simulink library "ammclib_bam_S32K3xx"  (R2016a)
settings: Solver=VariableStepAuto  SolverMode=SingleTasking  StartTime=0.0  StopTime=10.0  RelTol=1e-3
undefined symbols (not defined in the file or in its folder): a1, a2, ADCMaxError, autoCalcEn, b0, b1, b2, cfg, dgain, escale, f16A1, f16A2, f16ADCMaxError, f16B0, f16B1, f16B2, f16C1, f16CC1sc, f16CC1sc_D, f16CC1sc_Q, f16CC2sc, f16CC2sc_D, f16CC2sc_Q, f16DerivGain, f16EGain, f16FiltCoef, f16HystOff, f16HystOn, f16IGain, f16IntegGain, f16IntegGain_D, f16IntegGain_Q, f16IntegGainQ, f16Kd, f16KLs, f16Kq, f16KRs, f16Limit, f16LowerLimit, f16LowerLimit_D, f16LowerLimit_Q, f16LowerLimitQ, f16ModIndex, f16OutValOff, f16OutValOn, f16PropGain, f16PropGain_D, f16PropGain_Q, f16PropGainQ, f16RampDown, f16RampUp, f16UGain, f16UpperLimit, f16UpperLimit_D, f16UpperLimit_Q, f16UpperLimitQ, f16WIGain, f32A1, f32A2, f32ADCMaxError ... (+180)
(part 47 of 50)

== system ammclib_bam_S32K3xx/GFLIB/FLT/GFLIB_ControllerPIpAW_FLT ==
  fltInErr : Inport  OutDataTypeStr=single  SampleTime=SampleTime
  fltControllerPIpAWOut_preset : Inport  Port=2  OutDataTypeStr=single  SampleTime=SampleTime
  Reset : ResetPort  DisableCoverage=on
  GFLIB_ControllerPIpAW_SF : S-Function  FunctionName=GFLIB_ControllerPIpAW_SF_FLT  Parameters=showStates,resetStatesEnable,fltPropGain,fltIntegGain,fltLowerLimit,fltUpperLimit,pgain,igain,lowerLimit,upperLimit,autoCalcEn  SFunctionDeploymentMode=off  EnableBusSupport=off
  copyright : Subsystem
      mask Display: text(10,90,'FILE:');text(10,75,'DESRIPTION:');text(10,60,'COPYRIGHT:');text(10,45,'VERSION:');text(10,30,'DATE:')
  copyright2 : Subsystem
      mask Display: text(10,90,'GFLIB_ControllerPIpAW_BAM_FLT.slx');text(10,75,'Parallel form of a standard PI controller with anti-windup.');text(10,60,'NXP 2022');text(10,45,'1.0');text(10,30,'20-Apr-2022');
  fltInK_1 : Ground
  fltInK_1_Out : Terminator
  fltIntegGain : Ground
  fltIntegPartK_1 : Ground
  fltIntegPartK_1_Out : Terminator
  fltLowerLimit : Ground
  fltPropGain : Ground
  fltUpperLimit : Ground
  fltOut : Outport
  u16LimitFlag : Outport  Port=2
  wires:
  GFLIB_ControllerPIpAW_SF/4 -> fltInK_1_Out/1
  GFLIB_ControllerPIpAW_SF/3 -> fltIntegPartK_1_Out/1
  GFLIB_ControllerPIpAW_SF/2 -> u16LimitFlag/1
  GFLIB_ControllerPIpAW_SF/1 -> fltOut/1
  fltInK_1/1 -> GFLIB_ControllerPIpAW_SF/8
  fltIntegPartK_1/1 -> GFLIB_ControllerPIpAW_SF/7
  fltUpperLimit/1 -> GFLIB_ControllerPIpAW_SF/6
  fltLowerLimit/1 -> GFLIB_ControllerPIpAW_SF/5
  fltIntegGain/1 -> GFLIB_ControllerPIpAW_SF/4
  fltPropGain/1 -> GFLIB_ControllerPIpAW_SF/3
  fltControllerPIpAWOut_preset/1 -> GFLIB_ControllerPIpAW_SF/2
  fltInErr/1 -> GFLIB_ControllerPIpAW_SF/1

== system ammclib_bam_S32K3xx/GFLIB/FLT/GFLIB_ControllerPIp_FLT ==
  fltInErr : Inport  OutDataTypeStr=single  SampleTime=SampleTime
  fltControllerPIpOut_preset : Inport  Port=2  OutDataTypeStr=single  SampleTime=SampleTime
  Reset : ResetPort  DisableCoverage=on
  GFLIB_ControllerPIp_SF : S-Function  FunctionName=GFLIB_ControllerPIp_SF_FLT  Parameters=showStates,resetStatesEnable,fltPropGain,fltIntegGain,pgain,igain,autoCalcEn  SFunctionDeploymentMode=off  EnableBusSupport=off
  copyright : Subsystem
      mask Display: text(10,90,'FILE:');text(10,75,'DESRIPTION:');text(10,60,'COPYRIGHT:');text(10,45,'VERSION:');text(10,30,'DATE:')
  copyright2 : Subsystem
      mask Display: text(10,90,'GFLIB_ControllerPIp_BAM_FLT.slx');text(10,75,'Parallel form of a standard PI controller without anti-windup.');text(10,60,'NXP 2022');text(10,45,'1.0');text(10,30,'20-Apr-2022');
  fltInK_1 : Ground
  fltInK_1_Out : Terminator
  fltIntegGain : Ground
  fltIntegPartK_1 : Ground
  fltIntegPartK_1_Out : Terminator
  fltPropGain : Ground
  fltOut : Outport
  wires:
  GFLIB_ControllerPIp_SF/3 -> fltInK_1_Out/1
  GFLIB_ControllerPIp_SF/2 -> fltIntegPartK_1_Out/1
  GFLIB_ControllerPIp_SF/1 -> fltOut/1
  fltInK_1/1 -> GFLIB_ControllerPIp_SF/6
  fltIntegPartK_1/1 -> GFLIB_ControllerPIp_SF/5
  fltIntegGain/1 -> GFLIB_ControllerPIp_SF/4
  fltPropGain/1 -> GFLIB_ControllerPIp_SF/3
  fltControllerPIpOut_preset/1 -> GFLIB_ControllerPIp_SF/2
  fltInErr/1 -> GFLIB_ControllerPIp_SF/1

== system ammclib_bam_S32K3xx/GFLIB/FLT/GFLIB_ControllerPIrAW_FLT ==
  fltInErr : Inport  OutDataTypeStr=single  SampleTime=SampleTime
  fltControllerPIrAWOut_preset : Inport  Port=2  OutDataTypeStr=single  SampleTime=SampleTime
  Reset : ResetPort  DisableCoverage=on
  GFLIB_ControllerPIrAW_SF : S-Function  FunctionName=GFLIB_ControllerPIrAW_SF_FLT  Parameters=showStates,resetStatesEnable,fltUpperLimit,fltLowerLimit,fltCC1sc,fltCC2sc,intmethod,pgain,igain,upperLimit,lowerLimit,autoCalcEn  SFunctionDeploymentMode=off  EnableBusSupport=off
  copyright : Subsystem
      mask Display: text(10,90,'FILE:');text(10,75,'DESRIPTION:');text(10,60,'COPYRIGHT:');text(10,45,'VERSION:');text(10,30,'DATE:')
  copyright2 : Subsystem
      mask Display: text(10,90,'GFLIB_ControllerPIrAW_BAM_FLT.slx');text(10,75,'Recurrent form PI controller with anti-windup.');text(10,60,'NXP 2022');text(10,45,'1.0');text(10,30,'20-Apr-2022');
  fltAcc : Ground
  fltAcc_Out : Terminator
  fltCC1sc : Ground
  fltCC2sc : Ground
  fltInErrK1 : Ground
  fltInErrK1_Out : Terminator
  fltLowerLimit : Ground
  fltUpperLimit : Ground
  fltOut : Outport
  wires:
  GFLIB_ControllerPIrAW_SF/3 -> fltInErrK1_Out/1
  GFLIB_ControllerPIrAW_SF/2 -> fltAcc_Out/1
  GFLIB_ControllerPIrAW_SF/1 -> fltOut/1
  fltCC2sc/1 -> GFLIB_ControllerPIrAW_SF/8
  fltCC1sc/1 -> GFLIB_ControllerPIrAW_SF/7
  fltInErrK1/1 -> GFLIB_ControllerPIrAW_SF/6
  fltAcc/1 -> GFLIB_ControllerPIrAW_SF/5
  fltLowerLimit/1 -> GFLIB_ControllerPIrAW_SF/4
  fltUpperLimit/1 -> GFLIB_ControllerPIrAW_SF/3
  fltControllerPIrAWOut_preset/1 -> GFLIB_ControllerPIrAW_SF/2
  fltInErr/1 -> GFLIB_ControllerPIrAW_SF/1

== system ammclib_bam_S32K3xx/GFLIB/FLT/GFLIB_ControllerPIr_FLT ==
  fltInErr : Inport  OutDataTypeStr=single  SampleTime=SampleTime
  fltControllerPIrOut_preset : Inport  Port=2  OutDataTypeStr=single  SampleTime=SampleTime
  Reset : ResetPort  DisableCoverage=on
  GFLIB_ControllerPIr_SF : S-Function  FunctionName=GFLIB_ControllerPIr_SF_FLT  Parameters=showStates,resetStatesEnable,fltCC1sc,fltCC2sc,intmethod,pgain,igain,autoCalcEn  SFunctionDeploymentMode=off  EnableBusSupport=off
  copyright : Subsystem
      mask Display: text(10,90,'FILE:');text(10,75,'DESRIPTION:');text(10,60,'COPYRIGHT:');text(10,45,'VERSION:');text(10,30,'DATE:')
  copyright2 : Subsystem
      mask Display: text(10,90,'GFLIB_ControllerPIr_BAM_FLT.slx');text(10,75,'Recurrent form PI controller without anti-windup.');text(10,60,'NXP 2022');text(10,45,'1.0');text(10,30,'20-Apr-2022');
  fltAcc : Ground
  fltAcc_Out : Terminator
  fltCC1sc : Ground
  fltCC2sc : Ground
  fltInErrK1 : Ground
  fltInErrK1_Out : Terminator
  fltOut : Outport
  wires:
  GFLIB_ControllerPIr_SF/3 -> fltInErrK1_Out/1
  GFLIB_ControllerPIr_SF/2 -> fltAcc_Out/1
  GFLIB_ControllerPIr_SF/1 -> fltOut/1
  fltInErrK1/1 -> GFLIB_ControllerPIr_SF/6
  fltAcc/1 -> GFLIB_ControllerPIr_SF/5
  fltCC2sc/1 -> GFLIB_ControllerPIr_SF/4
  fltCC1sc/1 -> GFLIB_ControllerPIr_SF/3
  fltControllerPIrOut_preset/1 -> GFLIB_ControllerPIr_SF/2
  fltInErr/1 -> GFLIB_ControllerPIr_SF/1

== system ammclib_bam_S32K3xx/GFLIB/FLT/GFLIB_Cos_FLT ==
  fltIn : Inport  OutDataTypeStr=single
  GFLIB_Cos_SF : S-Function  FunctionName=GFLIB_Cos_SF_FLT  SFunctionDeploymentMode=off  EnableBusSupport=off
  copyright : Subsystem
      mask Display: text(10,90,'FILE:');text(10,75,'DESRIPTION:');text(10,60,'COPYRIGHT:');text(10,45,'VERSION:');text(10,30,'DATE:')
  copyright2 : Subsystem
      mask Display: text(10,90,'GFLIB_Cos_BAM_FLT.slx');text(10,75,'Cosine function');text(10,60,'NXP 2022');text(10,45,'1.0');text(10,30,'20-Apr-2022');
  fltOut : Outport
  wires:
  GFLIB_Cos_SF/1 -> fltOut/1
  fltIn/1 -> GFLIB_Cos_SF/1

== system ammclib_bam_S32K3xx/GFLIB/FLT/GFLIB_Hyst_FLT ==
  fltIn : Inport  OutDataTypeStr=single
  GFLIB_Hyst_SF : S-Function  FunctionName=GFLIB_Hyst_SF_FLT  Parameters=showStates,fltHystOn,fltHystOff,fltOutValOn,fltOutValOff  SFunctionDeploymentMode=off  EnableBusSupport=off
  copyright : Subsystem
      mask Display: text(10,90,'FILE:');text(10,75,'DESRIPTION:');text(10,60,'COPYRIGHT:');text(10,45,'VERSION:');text(10,30,'DATE:')
  copyright2 : Subsystem
      mask Display: text(10,90,'GFLIB_Hyst_BAM_FLT.slx');text(10,75,'Hysteresis function.');text(10,60,'NXP 2022');text(10,45,'1.0');text(10,30,'20-Apr-2022');
  fltHystOff : Ground
  fltHystOn : Ground
  fltOutState : Ground
  fltOutState_Out : Terminator
  fltOutValOff : Ground
  fltOutValOn : Ground
  fltOut : Outport
  wires:
  GFLIB_Hyst_SF/2 -> fltOutState_Out/1
  GFLIB_Hyst_SF/1 -> fltOut/1
  fltOutState/1 -> GFLIB_Hyst_SF/6
  fltOutValOff/1 -> GFLIB_Hyst_SF/5
  fltOutValOn/1 -> GFLIB_Hyst_SF/4
  fltHystOff/1 -> GFLIB_Hyst_SF/3
  fltHystOn/1 -> GFLIB_Hyst_SF/2
  fltIn/1 -> GFLIB_Hyst_SF/1

== system ammclib_bam_S32K3xx/GFLIB/FLT/GFLIB_IntegratorTR_FLT ==
  fltIn : Inport  OutDataTypeStr=single  SampleTime=SampleTime
  fltIntegratorTROut_preset : Inport  Port=2  OutDataTypeStr=single  SampleTime=SampleTime
  Reset : ResetPort  DisableCoverage=on
  GFLIB_IntegratorTR_SF : S-Function  FunctionName=GFLIB_IntegratorTR_SF_FLT  Parameters=showStates,resetStatesEnable,fltC1,autoCalcEn  SFunctionDeploymentMode=off  EnableBusSupport=off
  copyright : Subsystem
      mask Display: text(10,90,'FILE:');text(10,75,'DESRIPTION:');text(10,60,'COPYRIGHT:');text(10,45,'VERSION:');text(10,30,'DATE:')
  copyright2 : Subsystem
      mask Display: text(10,90,'GFLIB_IntegratorTR_BAM_FLT.slx');text(10,75,'Discrete-time integrator');text(10,60,'NXP 2022');text(10,45,'1.0');text(10,30,'20-Apr-2022');
  fltC1 : Ground
  fltInK1 : Ground
  fltInK1_Out : Terminator
  fltState : Ground
  fltState_Out : Terminator
  fltOut : Outport
  wires:
  GFLIB_IntegratorTR_SF/3 -> fltInK1_Out/1
  GFLIB_IntegratorTR_SF/2 -> fltState_Out/1
  GFLIB_IntegratorTR_SF/1 -> fltOut/1
  fltInK1/1 -> GFLIB_IntegratorTR_SF/5
  fltState/1 -> GFLIB_IntegratorTR_SF/4
  fltC1/1 -> GFLIB_IntegratorTR_SF/3
  fltIntegratorTROut_preset/1 -> GFLIB_IntegratorTR_SF/2
  fltIn/1 -> GFLIB_IntegratorTR_SF/1

== system ammclib_bam_S32K3xx/GFLIB/FLT/GFLIB_Limit_FLT ==
  fltIn : Inport  OutDataTypeStr=single
  GFLIB_Limit_SF : S-Function  FunctionName=GFLIB_Limit_SF_FLT  Parameters=showStates,fltLowerLimit,fltUpperLimit  SFunctionDeploymentMode=off  EnableBusSupport=off
  copyright : Subsystem
      mask Display: text(10,90,'FILE:');text(10,75,'DESRIPTION:');text(10,60,'COPYRIGHT:');text(10,45,'VERSION:');text(10,30,'DATE:')
  copyright2 : Subsystem
      mask Display: text(10,90,'GFLIB_Limit_BAM_FLT.slx');text(10,75,'Limit function.');text(10,60,'NXP 2022');text(10,45,'1.0');text(10,30,'20-Apr-2022');
  fltLowerLimit : Ground
  fltUpperLimit : Ground
  fltOut : Outport
  wires:
  GFLIB_Limit_SF/1 -> fltOut/1
  fltUpperLimit/1 -> GFLIB_Limit_SF/3
  fltLowerLimit/1 -> GFLIB_Limit_SF/2
  fltIn/1 -> GFLIB_Limit_SF/1

== system ammclib_bam_S32K3xx/GFLIB/FLT/GFLIB_Log10_FLT ==
  fltIn : Inport  OutDataTypeStr=single
  GFLIB_Log10_SF : S-Function  FunctionName=GFLIB_Log10_SF_FLT  SFunctionDeploymentMode=off  EnableBusSupport=off
  copyright : Subsystem
      mask Display: text(10,90,'FILE:');text(10,75,'DESRIPTION:');text(10,60,'COPYRIGHT:');text(10,45,'VERSION:');text(10,30,'DATE:')
  copyright2 : Subsystem
      mask Display: text(10,90,'GFLIB_Log10_BAM_FLT.slx');text(10,75,'Fast base-10 logarithm');text(10,60,'NXP 2022');text(10,45,'1.0');text(10,30,'20-Apr-2022');
  fltOut : Outport
  wires:
  GFLIB_Log10_SF/1 -> fltOut/1
  fltIn/1 -> GFLIB_Log10_SF/1

== system ammclib_bam_S32K3xx/GFLIB/FLT/GFLIB_LowerLimit_FLT ==
  fltIn : Inport  OutDataTypeStr=single
  GFLIB_LowerLimit_SF : S-Function  FunctionName=GFLIB_LowerLimit_SF_FLT  Parameters=showStates,fltLowerLimit  SFunctionDeploymentMode=off  EnableBusSupport=off
  copyright : Subsystem
      mask Display: text(10,90,'FILE:');text(10,75,'DESRIPTION:');text(10,60,'COPYRIGHT:');text(10,45,'VERSION:');text(10,30,'DATE:')
  copyright2 : Subsystem
      mask Display: text(10,90,'GFLIB_LowerLimit_BAM_FLT.slx');text(10,75,'Lower limit function.');text(10,60,'NXP 2022');text(10,45,'1.0');text(10,30,'20-Apr-2022');
  fltLowerLimit : Ground
  fltOut : Outport
  wires:
  GFLIB_LowerLimit_SF/1 -> fltOut/1
  fltLowerLimit/1 -> GFLIB_LowerLimit_SF/2
  fltIn/1 -> GFLIB_LowerLimit_SF/1

== system ammclib_bam_S32K3xx/GFLIB/FLT/GFLIB_Lut1D_FLT ==
  fltIn : Inport  OutDataTypeStr=single
  u32ShamOffset : Inport  Port=2  OutDataTypeStr=uint32
  GFLIB_Lut1D_SF : S-Function  FunctionName=GFLIB_Lut1D_SF_FLT  Parameters=pfltTable,s32MidIdx  SFunctionDeploymentMode=off  EnableBusSupport=off
  copyright : Subsystem
      mask Display: text(10,90,'FILE:');text(10,75,'DESRIPTION:');text(10,60,'COPYRIGHT:');text(10,45,'VERSION:');text(10,30,'DATE:')
  copyright2 : Subsystem
      mask Display: text(10,90,'GFLIB_Lut1D_BAM_FLT.slx');text(10,75,'One dimensional lookup table function');text(10,60,'NXP 2022');text(10,45,'1.0');text(10,30,'20-Apr-2022');
  fltOut : Outport
  wires:
  GFLIB_Lut1D_SF/1 -> fltOut/1
  u32ShamOffset/1 -> GFLIB_Lut1D_SF/2
  fltIn/1 -> GFLIB_Lut1D_SF/1

== system ammclib_bam_S32K3xx/GFLIB/FLT/GFLIB_Lut2D_FLT ==
  fltIn1 : Inport  OutDataTypeStr=single
  fltIn2 : Inport  Port=2  OutDataTypeStr=single
  u32ShamOffset1 : Inport  Port=3  OutDataTypeStr=uint32
  u32ShamOffset2 : Inport  Port=4  OutDataTypeStr=uint32
  GFLIB_Lut2D_SF : S-Function  FunctionName=GFLIB_Lut2D_SF_FLT  Parameters=pfltTable,s32MidIdx  SFunctionDeploymentMode=off  EnableBusSupport=off
  copyright : Subsystem
      mask Display: text(10,90,'FILE:');text(10,75,'DESRIPTION:');text(10,60,'COPYRIGHT:');text(10,45,'VERSION:');text(10,30,'DATE:')
  copyright2 : Subsystem
      mask Display: text(10,90,'GFLIB_Lut2D_BAM_FLT.slx');text(10,75,'Two dimensional lookup table function');text(10,60,'NXP 2022');text(10,45,'1.0');text(10,30,'20-Apr-2022');
  fltOut : Outport
  wires:
  GFLIB_Lut2D_SF/1 -> fltOut/1
  u32ShamOffset2/1 -> GFLIB_Lut2D_SF/4
  u32ShamOffset1/1 -> GFLIB_Lut2D_SF/3
  fltIn2/1 -> GFLIB_Lut2D_SF/2
  fltIn1/1 -> GFLIB_Lut2D_SF/1

== system ammclib_bam_S32K3xx/GFLIB/FLT/GFLIB_Ramp_FLT ==
  fltIn : Inport  OutDataTypeStr=single
  GFLIB_Ramp_SF : S-Function  FunctionName=GFLIB_Ramp_SF_FLT  Parameters=showStates,fltRampUp,fltRampDown  SFunctionDeploymentMode=off  EnableBusSupport=off
  copyright : Subsystem
      mask Display: text(10,90,'FILE:');text(10,75,'DESRIPTION:');text(10,60,'COPYRIGHT:');text(10,45,'VERSION:');text(10,30,'DATE:')
  copyright2 : Subsystem
      mask Display: text(10,90,'GFLIB_Ramp_BAM_FLT.slx');text(10,75,'Rate of change limiter - ramp function.');text(10,60,'NXP 2022');text(10,45,'1.0');text(10,30,'20-Apr-2022');
  fltRampDown : Ground
  fltRampUp : Ground
  fltState : Ground
  fltState_Out : Terminator
  fltOut : Outport
  wires:
  GFLIB_Ramp_SF/2 -> fltState_Out/1
  GFLIB_Ramp_SF/1 -> fltOut/1
  fltRampDown/1 -> GFLIB_Ramp_SF/4
  fltRampUp/1 -> GFLIB_Ramp_SF/3
  fltState/1 -> GFLIB_Ramp_SF/2
  fltIn/1 -> GFLIB_Ramp_SF/1

== system ammclib_bam_S32K3xx/GFLIB/FLT/GFLIB_Sign_FLT ==
  fltIn : Inport  OutDataTypeStr=single
  GFLIB_Sign_SF : S-Function  FunctionName=GFLIB_Sign_SF_FLT  SFunctionDeploymentMode=off  EnableBusSupport=off
  copyright : Subsystem
      mask Display: text(10,90,'FILE:');text(10,75,'DESRIPTION:');text(10,60,'COPYRIGHT:');text(10,45,'VERSION:');text(10,30,'DATE:')
  copyright2 : Subsystem
      mask Display: text(10,90,'GFLIB_Sign_BAM_FLT.slx');text(10,75,'Sign function.');text(10,60,'NXP 2022');text(10,45,'1.0');text(10,30,'20-Apr-2022');
  fltOut : Outport
  wires:
  GFLIB_Sign_SF/1 -> fltOut/1
  fltIn/1 -> GFLIB_Sign_SF/1

== system ammclib_bam_S32K3xx/GFLIB/FLT/GFLIB_SinCos_FLT ==
  fltIn : Inport  OutDataTypeStr=single
  GFLIB_SinCos_SF : S-Function  FunctionName=GFLIB_SinCos_SF_FLT  SFunctionDeploymentMode=off  EnableBusSupport=off
  copyright : Subsystem
      mask Display: text(10,90,'FILE:');text(10,75,'DESRIPTION:');text(10,60,'COPYRIGHT:');text(10,45,'VERSION:');text(10,30,'DATE:')
  copyright2 : Subsystem
      mask Display: text(10,90,'GFLIB_SinCos_BAM_FLT.slx');text(10,75,'Sine and cosine of the same argument');text(10,60,'NXP 2022');text(10,45,'1.0');text(10,30,'20-Apr-2022');
  pOut : Outport
  wires:
  GFLIB_SinCos_SF/1 -> pOut/1
  fltIn/1 -> GFLIB_SinCos_SF/1

== system ammclib_bam_S32K3xx/GFLIB/FLT/GFLIB_Sin_FLT ==
  fltIn : Inport  OutDataTypeStr=single
  GFLIB_Sin_SF : S-Function  FunctionName=GFLIB_Sin_SF_FLT  SFunctionDeploymentMode=off  EnableBusSupport=off
  copyright : Subsystem
      mask Display: text(10,90,'FILE:');text(10,75,'DESRIPTION:');text(10,60,'COPYRIGHT:');text(10,45,'VERSION:');text(10,30,'DATE:')
  copyright2 : Subsystem
      mask Display: text(10,90,'GFLIB_Sin_BAM_FLT.slx');text(10,75,'Sine function');text(10,60,'NXP 2022');text(10,45,'1.0');text(10,30,'20-Apr-2022');
  fltOut : Outport
  wires:
  GFLIB_Sin_SF/1 -> fltOut/1
  fltIn/1 -> GFLIB_Sin_SF/1

== system ammclib_bam_S32K3xx/GFLIB/FLT/GFLIB_Sqrt_FLT ==
  fltIn : Inport  OutDataTypeStr=single
  GFLIB_Sqrt_SF : S-Function  FunctionName=GFLIB_Sqrt_SF_FLT  SFunctionDeploymentMode=off  EnableBusSupport=off
  copyright : Subsystem
      mask Display: text(10,90,'FILE:');text(10,75,'DESRIPTION:');text(10,60,'COPYRIGHT:');text(10,45,'VERSION:');text(10,30,'DATE:')
  copyright2 : Subsystem
      mask Display: text(10,90,'GFLIB_Sqrt_BAM_FLT.slx');text(10,75,'Square root approximation.');text(10,60,'NXP 2022');text(10,45,'1.0');text(10,30,'20-Apr-2022');
  fltOut : Outport
  wires:
  GFLIB_Sqrt_SF/1 -> fltOut/1
  fltIn/1 -> GFLIB_Sqrt_SF/1

== system ammclib_bam_S32K3xx/GFLIB/FLT/GFLIB_Tan_FLT ==
  fltIn : Inport  OutDataTypeStr=single
  GFLIB_Tan_SF : S-Function  FunctionName=GFLIB_Tan_SF_FLT  SFunctionDeploymentMode=off  EnableBusSupport=off
  copyright : Subsystem
      mask Display: text(10,90,'FILE:');text(10,75,'DESRIPTION:');text(10,60,'COPYRIGHT:');text(10,45,'VERSION:');text(10,30,'DATE:')
  copyright2 : Subsystem
      mask Display: text(10,90,'GFLIB_Tan_BAM_FLT.slx');text(10,75,'Trigonometric tangent function');text(10,60,'NXP 2022');text(10,45,'1.0');text(10,30,'20-Apr-2022');
  fltOut : Outport
  wires:
  GFLIB_Tan_SF/1 -> fltOut/1
  fltIn/1 -> GFLIB_Tan_SF/1

== system ammclib_bam_S32K3xx/GFLIB/FLT/GFLIB_UpperLimit_FLT ==
  fltIn : Inport  OutDataTypeStr=single
  GFLIB_UpperLimit_SF : S-Function  FunctionName=GFLIB_UpperLimit_SF_FLT  Parameters=showStates,fltUpperLimit  SFunctionDeploymentMode=off  EnableBusSupport=off
  copyright : Subsystem
      mask Display: text(10,90,'FILE:');text(10,75,'DESRIPTION:');text(10,60,'COPYRIGHT:');text(10,45,'VERSION:');text(10,30,'DATE:')
  copyright2 : Subsystem
      mask Display: text(10,90,'GFLIB_UpperLimit_BAM_FLT.slx');text(10,75,'Upper limit function.');text(10,60,'NXP 2022');text(10,45,'1.0');text(10,30,'20-Apr-2022');
  fltUpperLimit : Ground
  fltOut : Outport
  wires:
  GFLIB_UpperLimit_SF/1 -> fltOut/1
  fltUpperLimit/1 -> GFLIB_UpperLimit_SF/2
  fltIn/1 -> GFLIB_UpperLimit_SF/1

== system ammclib_bam_S32K3xx/GFLIB/FLT/GFLIB_VLog10_FLT ==
  pIn : Inport  OutDataTypeStr=single
  GFLIB_VLog10_SF : S-Function  FunctionName=GFLIB_VLog10_SF_FLT  SFunctionDeploymentMode=off  EnableBusSupport=off
  copyright : Subsystem
      mask Display: text(10,90,'FILE:');text(10,75,'DESRIPTION:');text(10,60,'COPYRIGHT:');text(10,45,'VERSION:');text(10,30,'DATE:')
  copyright2 : Subsystem
      mask Display: text(10,90,'GFLIB_VLog10_BAM_FLT.slx');text(10,75,'Vector base-10 logarithm');text(10,60,'NXP 2022');text(10,45,'1.0');text(10,30,'20-Apr-2022');
  pOut : Outport
  wires:
  GFLIB_VLog10_SF/1 -> pOut/1
  pIn/1 -> GFLIB_VLog10_SF/1

== system ammclib_bam_S32K3xx/GFLIB/FLT/GFLIB_VMin_FLT ==
  pIn : Inport  OutDataTypeStr=single
  GFLIB_VMin_SF : S-Function  FunctionName=GFLIB_VMin_SF_FLT  SFunctionDeploymentMode=off  EnableBusSupport=off
  copyright : Subsystem
      mask Display: text(10,90,'FILE:');text(10,75,'DESRIPTION:');text(10,60,'COPYRIGHT:');text(10,45,'VERSION:');text(10,30,'DATE:')
  copyright2 : Subsystem
      mask Display: text(10,90,'GFLIB_VMin_BAM_FLT.slx');text(10,75,'Vector minimum');text(10,60,'NXP 2022');text(10,45,'1.0');text(10,30,'20-Apr-2022');
  IndexOfMinimum : Outport
  wires:
  GFLIB_VMin_SF/1 -> IndexOfMinimum/1
  pIn/1 -> GFLIB_VMin_SF/1

== system ammclib_bam_S32K3xx/GFLIB/FLT/GFLIB_VectorLimit_FLT ==
  pIn : Inport  OutDataTypeStr=Bus: SWLIBS_2Syst_FLT  BusOutputAsStruct=on
  GFLIB_VectorLimit_SF : S-Function  FunctionName=GFLIB_VectorLimit_SF_FLT  Parameters=showStates,fltLimit  SFunctionDeploymentMode=off  EnableBusSupport=off
  copyright : Subsystem
      mask Display: text(10,90,'FILE:');text(10,75,'DESRIPTION:');text(10,60,'COPYRIGHT:');text(10,45,'VERSION:');text(10,30,'DATE:')
  copyright2 : Subsystem
      mask Display: text(10,90,'GFLIB_VectorLimit_BAM_FLT.slx');text(10,75,'Vector Limit function.');text(10,60,'NXP 2022');text(10,45,'1.0');text(10,30,'20-Apr-2022');
  fltLimit : Ground
  bFlag : Outport
  pOut : Outport  Port=2
  wires:
  GFLIB_VectorLimit_SF/2 -> pOut/1
  GFLIB_VectorLimit_SF/1 -> bFlag/1
  fltLimit/1 -> GFLIB_VectorLimit_SF/2
  pIn/1 -> GFLIB_VectorLimit_SF/1

== system ammclib_bam_S32K3xx/GMCLIB/F16/GMCLIB_BetaProjection3Ph_F16 ==
  pIn : Inport  OutDataTypeStr=Bus: SWLIBS_3Syst_F16  BusOutputAsStruct=on
  GMCLIB_BetaProjection3Ph_SF : S-Function  FunctionName=GMCLIB_BetaProjection3Ph_SF_F16  SFunctionDeploymentMode=off  EnableBusSupport=off
  copyright : Subsystem
      mask Display: text(10,90,'FILE:');text(10,75,'DESRIPTION:');text(10,60,'COPYRIGHT:');text(10,45,'VERSION:');text(10,30,'DATE:')
  copyright2 : Subsystem
      mask Display: text(10,90,'GMCLIB_BetaProjection3Ph_BAM_F16.slx');text(10,75,'3-phase Beta-projection transformation.');text(10,60,'NXP 2022');text(10,45,'1.0');text(10,30,'20-Apr-2022');
  pOut : Outport
  wires:
  GMCLIB_BetaProjection3Ph_SF/1 -> pOut/1
  pIn/1 -> GMCLIB_BetaProjection3Ph_SF/1

== system ammclib_bam_S32K3xx/GMCLIB/F16/GMCLIB_BetaProjection_F16 ==
  pIn : Inport  OutDataTypeStr=Bus: SWLIBS_3Syst_F16  BusOutputAsStruct=on
  GMCLIB_BetaProjection_SF : S-Function  FunctionName=GMCLIB_BetaProjection_SF_F16  SFunctionDeploymentMode=off  EnableBusSupport=off
  copyright : Subsystem
      mask Display: text(10,90,'FILE:');text(10,75,'DESRIPTION:');text(10,60,'COPYRIGHT:');text(10,45,'VERSION:');text(10,30,'DATE:')
  copyright2 : Subsystem
      mask Display: text(10,90,'GMCLIB_BetaProjection_BAM_F16.slx');text(10,75,'Beta Projection transformation.');text(10,60,'NXP 2022');text(10,45,'1.0');text(10,30,'20-Apr-2022');
  pOut : Outport
  wires:
  GMCLIB_BetaProjection_SF/1 -> pOut/1
  pIn/1 -> GMCLIB_BetaProjection_SF/1

== system ammclib_bam_S32K3xx/GMCLIB/F16/GMCLIB_Clark6Ph_F16 ==
  pIn : Inport  OutDataTypeStr=Bus: SWLIBS_6Syst_F16  BusOutputAsStruct=on
  GMCLIB_Clark6Ph_SF : S-Function  FunctionName=GMCLIB_Clark6Ph_SF_F16  Parameters=f16WindingShift  SFunctionDeploymentMode=off  EnableBusSupport=off
  copyright : Subsystem
      mask Display: text(10,90,'FILE:');text(10,75,'DESRIPTION:');text(10,60,'COPYRIGHT:');text(10,45,'VERSION:');text(10,30,'DATE:')
  copyright2 : Subsystem
      mask Display: text(10,90,'GMCLIB_Clark6Ph_BAM_F16.slx');text(10,75,'Direct 6-phase Clark transformation.');text(10,60,'NXP 2022');text(10,45,'1.0');text(10,30,'20-Apr-2022');
  pOut : Outport
  wires:
  GMCLIB_Clark6Ph_SF/1 -> pOut/1
  pIn/1 -> GMCLIB_Clark6Ph_SF/1

== system ammclib_bam_S32K3xx/GMCLIB/F16/GMCLIB_ClarkInv6Ph_F16 ==
  pIn : Inport  OutDataTypeStr=Bus: SWLIBS_2Syst_F16  BusOutputAsStruct=on
  GMCLIB_ClarkInv6Ph_SF : S-Function  FunctionName=GMCLIB_ClarkInv6Ph_SF_F16  Parameters=f16WindingShift  SFunctionDeploymentMode=off  EnableBusSupport=off
  copyright : Subsystem
      mask Display: text(10,90,'FILE:');text(10,75,'DESRIPTION:');text(10,60,'COPYRIGHT:');text(10,45,'VERSION:');text(10,30,'DATE:')
  copyright2 : Subsystem
      mask Display: text(10,90,'GMCLIB_ClarkInv6Ph_BAM_F16.slx');text(10,75,'Inverse Clarke transform for six-phase systems.');text(10,60,'NXP 2022');text(10,45,'1.0');text(10,30,'20-Apr-2022');
  pOut : Outport
  wires:
  GMCLIB_ClarkInv6Ph_SF/1 -> pOut/1
  pIn/1 -> GMCLIB_ClarkInv6Ph_SF/1

== system ammclib_bam_S32K3xx/GMCLIB/F16/GMCLIB_ClarkInv_F16 ==
  pIn : Inport  OutDataTypeStr=Bus: SWLIBS_2Syst_F16  BusOutputAsStruct=on
  GMCLIB_ClarkInv_SF : S-Function  FunctionName=GMCLIB_ClarkInv_SF_F16  SFunctionDeploymentMode=off  EnableBusSupport=off
  copyright : Subsystem
      mask Display: text(10,90,'FILE:');text(10,75,'DESRIPTION:');text(10,60,'COPYRIGHT:');text(10,45,'VERSION:');text(10,30,'DATE:')
  copyright2 : Subsystem
      mask Display: text(10,90,'GMCLIB_ClarkInv_BAM_F16.slx');text(10,75,'Inverse Clarke transformation');text(10,60,'NXP 2022');text(10,45,'1.0');text(10,30,'20-Apr-2022');
  pOut : Outport
  wires:
  GMCLIB_ClarkInv_SF/1 -> pOut/1
  pIn/1 -> GMCLIB_ClarkInv_SF/1

== system ammclib_bam_S32K3xx/GMCLIB/F16/GMCLIB_Clark_F16 ==
  pIn : Inport  OutDataTypeStr=Bus: SWLIBS_3Syst_F16  BusOutputAsStruct=on
  GMCLIB_Clark_SF : S-Function  FunctionName=GMCLIB_Clark_SF_F16  SFunctionDeploymentMode=off  EnableBusSupport=off
  copyright : Subsystem
      mask Display: text(10,90,'FILE:');text(10,75,'DESRIPTION:');text(10,60,'COPYRIGHT:');text(10,45,'VERSION:');text(10,30,'DATE:')
  copyright2 : Subsystem
      mask Display: text(10,90,'GMCLIB_Clark_BAM_F16.slx');text(10,75,'Clarke transformation.');text(10,60,'NXP 2022');text(10,45,'1.0');text(10,30,'20-Apr-2022');
  pOut : Outport
  wires:
  GMCLIB_Clark_SF/1 -> pOut/1
  pIn/1 -> GMCLIB_Clark_SF/1

== system ammclib_bam_S32K3xx/GMCLIB/F16/GMCLIB_DecouplingPMSM_F16 ==
  pUdq : Inport  OutDataTypeStr=Bus: SWLIBS_2Syst_F16  BusOutputAsStruct=on
  pIdq : Inport  Port=2  OutDataTypeStr=Bus: SWLIBS_2Syst_F16  BusOutputAsStruct=on
  f16AngularVel : Inport  Port=3  OutDataTypeStr=int16
  GMCLIB_DecouplingPMSM_SF : S-Function  FunctionName=GMCLIB_DecouplingPMSM_SF_F16  Parameters=showStates,f16Kd,s16KdShift,f16Kq,s16KqShift  SFunctionDeploymentMode=off  EnableBusSupport=off
  copyright : Subsystem
      mask Display: text(10,90,'FILE:');text(10,75,'DESRIPTION:');text(10,60,'COPYRIGHT:');text(10,45,'VERSION:');text(10,30,'DATE:')
  copyright2 : Subsystem
      mask Display: text(10,90,'GMCLIB_DecouplingPMSM_BAM_F16.slx');text(10,75,'Decoupling of d and q axis of PMSM model.');text(10,60,'NXP 2022');text(10,45,'1.0');text(10,30,'20-Apr-2022');
  f16Kd : Ground
  f16Kq : Ground
  s16KdShift : Ground
  s16KqShift : Ground
  pUdqDec : Outport
  wires:
  GMCLIB_DecouplingPMSM_SF/1 -> pUdqDec/1
  s16KqShift/1 -> GMCLIB_DecouplingPMSM_SF/7
  f16Kq/1 -> GMCLIB_DecouplingPMSM_SF/6
  s16KdShift/1 -> GMCLIB_DecouplingPMSM_SF/5
  f16Kd/1 -> GMCLIB_DecouplingPMSM_SF/4
  f16AngularVel/1 -> GMCLIB_DecouplingPMSM_SF/3
  pIdq/1 -> GMCLIB_DecouplingPMSM_SF/2
  pUdq/1 -> GMCLIB_DecouplingPMSM_SF/1

== system ammclib_bam_S32K3xx/GMCLIB/F16/GMCLIB_DoubleSwitching_F16 ==
  pInPwm : Inport  OutDataTypeStr=Bus: SWLIBS_3Syst_F16  BusOutputAsStruct=on
  u16Sector : Inport  Port=2  OutDataTypeStr=uint16
  pParam : Inport  Port=3  OutDataTypeStr=Bus: GMCLIB_DOUBLESWITCHING_T_F16  BusOutputAsStruct=on
  GMCLIB_DoubleSwitching_SF : S-Function  FunctionName=GMCLIB_DoubleSwitching_SF_F16  SFunctionDeploymentMode=off  EnableBusSupport=off
  copyright : Subsystem
      mask Display: text(10,90,'FILE:');text(10,75,'DESRIPTION:');text(10,60,'COPYRIGHT:');text(10,45,'VERSION:');text(10,30,'DATE:')
  copyright2 : Subsystem
      mask Display: text(10,90,'GMCLIB_DoubleSwitching_BAM_F16.slx');text(10,75,'DoubleSwitching algorithm.');text(10,60,'NXP 2022');text(10,45,'1.0');text(10,30,'20-Apr-2022');
  pOutEdges : Outport
  pOutTriggers : Outport  Port=2
  wires:
  GMCLIB_DoubleSwitching_SF/2 -> pOutTriggers/1
  GMCLIB_DoubleSwitching_SF/1 -> pOutEdges/1
  pParam/1 -> GMCLIB_DoubleSwitching_SF/3
  u16Sector/1 -> GMCLIB_DoubleSwitching_SF/2
  pInPwm/1 -> GMCLIB_DoubleSwitching_SF/1

== system ammclib_bam_S32K3xx/GMCLIB/F16/GMCLIB_ElimDcBusRip_F16 ==
  pIn : Inport  OutDataTypeStr=Bus: SWLIBS_2Syst_F16  BusOutputAsStruct=on
  f16ArgDcBusMsr : Inport  Port=2  OutDataTypeStr=int16
  GMCLIB_ElimDcBusRip_SF : S-Function  FunctionName=GMCLIB_ElimDcBusRip_SF_F16  Parameters=showStates,f16ModIndex  SFunctionDeploymentMode=off  EnableBusSupport=off
  copyright : Subsystem
      mask Display: text(10,90,'FILE:');text(10,75,'DESRIPTION:');text(10,60,'COPYRIGHT:');text(10,45,'VERSION:');text(10,30,'DATE:')
  copyright2 : Subsystem
      mask Display: text(10,90,'GMCLIB_ElimDcBusRip_BAM_F16.slx');text(10,75,'DC Bus voltage ripple elimination function.');text(10,60,'NXP 2022');text(10,45,'1.0');text(10,30,'20-Apr-2022');
  f16ModIndex : Ground
  pOut : Outport
  wires:
  GMCLIB_ElimDcBusRip_SF/1 -> pOut/1
  f16ModIndex/1 -> GMCLIB_ElimDcBusRip_SF/3
  f16ArgDcBusMsr/1 -> GMCLIB_ElimDcBusRip_SF/2
  pIn/1 -> GMCLIB_ElimDcBusRip_SF/1

== system ammclib_bam_S32K3xx/GMCLIB/F16/GMCLIB_ParkInv_F16 ==
  pInAngle : Inport  OutDataTypeStr=Bus: SWLIBS_2Syst_F16  BusOutputAsStruct=on
  pIn : Inport  Port=2  OutDataTypeStr=Bus: SWLIBS_2Syst_F16  BusOutputAsStruct=on
  GMCLIB_ParkInv_SF : S-Function  FunctionName=GMCLIB_ParkInv_SF_F16  SFunctionDeploymentMode=off  EnableBusSupport=off
  copyright : Subsystem
      mask Display: text(10,90,'FILE:');text(10,75,'DESRIPTION:');text(10,60,'COPYRIGHT:');text(10,45,'VERSION:');text(10,30,'DATE:')
  copyright2 : Subsystem
      mask Display: text(10,90,'GMCLIB_ParkInv_BAM_F16.slx');text(10,75,'Inverse Park transformation.');text(10,60,'NXP 2022');text(10,45,'1.0');text(10,30,'20-Apr-2022');
  pOut : Outport
  wires:
  GMCLIB_ParkInv_SF/1 -> pOut/1
  pIn/1 -> GMCLIB_ParkInv_SF/2
  pInAngle/1 -> GMCLIB_ParkInv_SF/1

== system ammclib_bam_S32K3xx/GMCLIB/F16/GMCLIB_Park_F16 ==
  pInAngle : Inport  OutDataTypeStr=Bus: SWLIBS_2Syst_F16  BusOutputAsStruct=on
  pIn : Inport  Port=2  OutDataTypeStr=Bus: SWLIBS_2Syst_F16  BusOutputAsStruct=on
  GMCLIB_Park_SF : S-Function  FunctionName=GMCLIB_Park_SF_F16  SFunctionDeploymentMode=off  EnableBusSupport=off
  copyright : Subsystem
      mask Display: text(10,90,'FILE:');text(10,75,'DESRIPTION:');text(10,60,'COPYRIGHT:');text(10,45,'VERSION:');text(10,30,'DATE:')
  copyright2 : Subsystem
      mask Display: text(10,90,'GMCLIB_Park_BAM_F16.slx');text(10,75,'Park transformation.');text(10,60,'NXP 2022');text(10,45,'1.0');text(10,30,'20-Apr-2022');
  pOut : Outport
  wires:
  GMCLIB_Park_SF/1 -> pOut/1
  pIn/1 -> GMCLIB_Park_SF/2
  pInAngle/1 -> GMCLIB_Park_SF/1

== system ammclib_bam_S32K3xx/GMCLIB/F16/GMCLIB_PwmIct_F16 ==
  pIn : Inport  OutDataTypeStr=Bus: SWLIBS_2Syst_F16  BusOutputAsStruct=on
  GMCLIB_PwmIct_SF : S-Function  FunctionName=GMCLIB_PwmIct_SF_F16  SFunctionDeploymentMode=off  EnableBusSupport=off
  copyright : Subsystem
      mask Display: text(10,90,'FILE:');text(10,75,'DESRIPTION:');text(10,60,'COPYRIGHT:');text(10,45,'VERSION:');text(10,30,'DATE:')
  copyright2 : Subsystem
      mask Display: text(10,90,'GMCLIB_PwmIct_BAM_F16.slx');text(10,75,'General Sinusoidal PWM.');text(10,60,'NXP 2022');text(10,45,'1.0');text(10,30,'20-Apr-2022');
  u16Sector : Outport
  pOut : Outport  Port=2
  wires:
  GMCLIB_PwmIct_SF/2 -> pOut/1
  GMCLIB_PwmIct_SF/1 -> u16Sector/1
  pIn/1 -> GMCLIB_PwmIct_SF/1

== system ammclib_bam_S32K3xx/GMCLIB/F16/GMCLIB_SvmSci_F16 ==
  pIn : Inport  OutDataTypeStr=Bus: SWLIBS_2Syst_F16  BusOutputAsStruct=on
  GMCLIB_SvmSci_SF : S-Function  FunctionName=GMCLIB_SvmSci_SF_F16  SFunctionDeploymentMode=off  EnableBusSupport=off
  copyright : Subsystem
      mask Display: text(10,90,'FILE:');text(10,75,'DESRIPTION:');text(10,60,'COPYRIGHT:');text(10,45,'VERSION:');text(10,30,'DATE:')
  copyright2 : Subsystem
      mask Display: text(10,90,'GMCLIB_SvmSci_BAM_F16.slx');text(10,75,'General Sinusoidal Modulation with Injection of Third Harmonic.');text(10,60,'NXP 2022');text(10,45,'1.0');text(10,30,'20-Apr-2022');
  u16Sector : Outport
  pOut : Outport  Port=2
  wires:
  GMCLIB_SvmSci_SF/2 -> pOut/1
  GMCLIB_SvmSci_SF/1 -> u16Sector/1
  pIn/1 -> GMCLIB_SvmSci_SF/1

== system ammclib_bam_S32K3xx/GMCLIB/F16/GMCLIB_SvmStd6Ph_F16 ==
  pIn : Inport  OutDataTypeStr=Bus: SWLIBS_2Syst_F16  BusOutputAsStruct=on
  GMCLIB_SvmStd6Ph_SF : S-Function  FunctionName=GMCLIB_SvmStd6Ph_SF_F16  Parameters=f16WindingShift  SFunctionDeploymentMode=off  EnableBusSupport=off
  copyright : Subsystem
      mask Display: text(10,90,'FILE:');text(10,75,'DESRIPTION:');text(10,60,'COPYRIGHT:');text(10,45,'VERSION:');text(10,30,'DATE:')
  copyright2 : Subsystem
      mask Display: text(10,90,'GMCLIB_SvmStd6Ph_BAM_F16.slx');text(10,75,'Six-phase Space Vector Modulation.');text(10,60,'NXP 2022');text(10,45,'1.0');text(10,30,'20-Apr-2022');
  pOut : Outport
  pOutSector : Outport  Port=2
  wires:
  GMCLIB_SvmStd6Ph_SF/2 -> pOutSector/1
  GMCLIB_SvmStd6Ph_SF/1 -> pOut/1
  pIn/1 -> GMCLIB_SvmStd6Ph_SF/1

== system ammclib_bam_S32K3xx/GMCLIB/F16/GMCLIB_SvmStd_F16 ==
  pIn : Inport  OutDataTypeStr=Bus: SWLIBS_2Syst_F16  BusOutputAsStruct=on
  GMCLIB_SvmStd_SF : S-Function  FunctionName=GMCLIB_SvmStd_SF_F16  SFunctionDeploymentMode=off  EnableBusSupport=off
  copyright : Subsystem
      mask Display: text(10,90,'FILE:');text(10,75,'DESRIPTION:');text(10,60,'COPYRIGHT:');text(10,45,'VERSION:');text(10,30,'DATE:')
  copyright2 : Subsystem
      mask Display: text(10,90,'GMCLIB_SvmStd_BAM_F16.slx');text(10,75,'Standard Space Vector Modulation.');text(10,60,'NXP 2022');text(10,45,'1.0');text(10,30,'20-Apr-2022');
  u16Sector : Outport
  pOut : Outport  Port=2
  wires:
  GMCLIB_SvmStd_SF/2 -> pOut/1
  GMCLIB_SvmStd_SF/1 -> u16Sector/1
  pIn/1 -> GMCLIB_SvmStd_SF/1

== system ammclib_bam_S32K3xx/GMCLIB/F16/GMCLIB_SvmU0n_F16 ==
  pIn : Inport  OutDataTypeStr=Bus: SWLIBS_2Syst_F16  BusOutputAsStruct=on
  GMCLIB_SvmU0n_SF : S-Function  FunctionName=GMCLIB_SvmU0n_SF_F16  SFunctionDeploymentMode=off  EnableBusSupport=off
  copyright : Subsystem
      mask Display: text(10,90,'FILE:');text(10,75,'DESRIPTION:');text(10,60,'COPYRIGHT:');text(10,45,'VERSION:');text(10,30,'DATE:')
  copyright2 : Subsystem
      mask Display: text(10,90,'GMCLIB_SvmU0n_BAM_F16.slx');text(10,75,'Special Space Vector Modulation with O_000 Nulls.');text(10,60,'NXP 2022');text(10,45,'1.0');text(10,30,'20-Apr-2022');
  u16Sector : Outport
  pOut : Outport  Port=2
  wires:
  GMCLIB_SvmU0n_SF/2 -> pOut/1
  GMCLIB_SvmU0n_SF/1 -> u16Sector/1
  pIn/1 -> GMCLIB_SvmU0n_SF/1

== system ammclib_bam_S32K3xx/GMCLIB/F16/GMCLIB_SvmU7n_F16 ==
  pIn : Inport  OutDataTypeStr=Bus: SWLIBS_2Syst_F16  BusOutputAsStruct=on
  GMCLIB_SvmU7n_SF : S-Function  FunctionName=GMCLIB_SvmU7n_SF_F16  SFunctionDeploymentMode=off  EnableBusSupport=off
  copyright : Subsystem
      mask Display: text(10,90,'FILE:');text(10,75,'DESRIPTION:');text(10,60,'COPYRIGHT:');text(10,45,'VERSION:');text(10,30,'DATE:')
  copyright2 : Subsystem
      mask Display: text(10,90,'GMCLIB_SvmU7n_BAM_F16.slx');text(10,75,'Special Space Vector Modulation with O_111 Ones.');text(10,60,'NXP 2022');text(10,45,'1.0');text(10,30,'20-Apr-2022');
  u16Sector : Outport
  pOut : Outport  Port=2
  wires:
  GMCLIB_SvmU7n_SF/2 -> pOut/1
  GMCLIB_SvmU7n_SF/1 -> u16Sector/1
  pIn/1 -> GMCLIB_SvmU7n_SF/1

== system ammclib_bam_S32K3xx/GMCLIB/F16/GMCLIB_VRot_F16 ==
  f16InVec : Inport  OutDataTypeStr=Bus: SWLIBS_2Syst_F16  BusOutputAsStruct=on
  f16Angle : Inport  Port=2  OutDataTypeStr=int16
  GMCLIB_VRot_SF : S-Function  FunctionName=GMCLIB_VRot_SF_F16  SFunctionDeploymentMode=off  EnableBusSupport=off
  copyright : Subsystem
      mask Display: text(10,90,'FILE:');text(10,75,'DESRIPTION:');text(10,60,'COPYRIGHT:');text(10,45,'VERSION:');text(10,30,'DATE:')
  copyright2 : Subsystem
      mask Display: text(10,90,'GMCLIB_VRot_BAM_F16.slx');text(10,75,'Vector rotation.');text(10,60,'NXP 2022');text(10,45,'1.0');text(10,30,'20-Apr-2022');
  f16OutVec : Outport
  wires:
  GMCLIB_VRot_SF/1 -> f16OutVec/1
  f16Angle/1 -> GMCLIB_VRot_SF/2
  f16InVec/1 -> GMCLIB_VRot_SF/1

== system ammclib_bam_S32K3xx/GMCLIB/F16/GMCLIB_VUnit_F16 ==
  f16InVec : Inport  OutDataTypeStr=Bus: SWLIBS_2Syst_F16  BusOutputAsStruct=on
  GMCLIB_VUnit_SF : S-Function  FunctionName=GMCLIB_VUnit_SF_F16  SFunctionDeploymentMode=off  EnableBusSupport=off
  copyright : Subsystem
      mask Display: text(10,90,'FILE:');text(10,75,'DESRIPTION:');text(10,60,'COPYRIGHT:');text(10,45,'VERSION:');text(10,30,'DATE:')
  copyright2 : Subsystem
      mask Display: text(10,90,'GMCLIB_VUnit_BAM_F16.slx');text(10,75,'Vector normalization.');text(10,60,'NXP 2022');text(10,45,'1.0');text(10,30,'20-Apr-2022');
  f16OutVec : Outport
  wires:
  GMCLIB_VUnit_SF/1 -> f16OutVec/1
  f16InVec/1 -> GMCLIB_VUnit_SF/1

== system ammclib_bam_S32K3xx/GMCLIB/F16/GMCLIB_Vmag2coord_F16 ==
  f16InMag : Inport  OutDataTypeStr=int16
  f16InCoord : Inport  Port=2  OutDataTypeStr=int16
  GMCLIB_Vmag2coord_SF : S-Function  FunctionName=GMCLIB_Vmag2coord_SF_F16  SFunctionDeploymentMode=off  EnableBusSupport=off
  copyright : Subsystem
      mask Display: text(10,90,'FILE:');text(10,75,'DESRIPTION:');text(10,60,'COPYRIGHT:');text(10,45,'VERSION:');text(10,30,'DATE:')
  copyright2 : Subsystem
      mask Display: text(10,90,'GMCLIB_Vmag2coord_BAM_F16.slx');text(10,75,'Calculation of the coordinate out of the magnitute and second coordinate.');text(10,60,'NXP 2022');text(10,45,'1.0');text(10,30,'20-Apr-2022');
  f16OutCoord : Outport
  wires:
  GMCLIB_Vmag2coord_SF/1 -> f16OutCoord/1
  f16InCoord/1 -> GMCLIB_Vmag2coord_SF/2
  f16InMag/1 -> GMCLIB_Vmag2coord_SF/1

== system ammclib_bam_S32K3xx/GMCLIB/F16/GMCLIB_Vpol2xy_F16 ==
  f16InVec : Inport  OutDataTypeStr=Bus: SWLIBS_2Syst_F16  BusOutputAsStruct=on
  GMCLIB_Vpol2xy_SF : S-Function  FunctionName=GMCLIB_Vpol2xy_SF_F16  SFunctionDeploymentMode=off  EnableBusSupport=off
  copyright : Subsystem
      mask Display: text(10,90,'FILE:');text(10,75,'DESRIPTION:');text(10,60,'COPYRIGHT:');text(10,45,'VERSION:');text(10,30,'DATE:')
  copyright2 : Subsystem
      mask Display: text(10,90,'GMCLIB_Vpol2xy_BAM_F16.slx');text(10,75,'Transformation of polar coordinate system to Cartesian.');text(10,60,'NXP 2022');text(10,45,'1.0');text(10,30,'20-Apr-2022');
  f16OutVec : Outport
  wires:
  GMCLIB_Vpol2xy_SF/1 -> f16OutVec/1
  f16InVec/1 -> GMCLIB_Vpol2xy_SF/1

== system ammclib_bam_S32K3xx/GMCLIB/F16/GMCLIB_Vxy2pol_F16 ==
  f16InVec : Inport  OutDataTypeStr=Bus: SWLIBS_2Syst_F16  BusOutputAsStruct=on
  GMCLIB_Vxy2pol_SF : S-Function  FunctionName=GMCLIB_Vxy2pol_SF_F16  SFunctionDeploymentMode=off  EnableBusSupport=off
  copyright : Subsystem
      mask Display: text(10,90,'FILE:');text(10,75,'DESRIPTION:');text(10,60,'COPYRIGHT:');text(10,45,'VERSION:');text(10,30,'DATE:')
  copyright2 : Subsystem
      mask Display: text(10,90,'GMCLIB_Vxy2pol_BAM_F16.slx');text(10,75,'Transformation of Cartesian coordinate system to polar.');text(10,60,'NXP 2022');text(10,45,'1.0');text(10,30,'20-Apr-2022');
  f16OutVec : Outport
  wires:
  GMCLIB_Vxy2pol_SF/1 -> f16OutVec/1
  f16InVec/1 -> GMCLIB_Vxy2pol_SF/1

== system ammclib_bam_S32K3xx/GMCLIB/F32/GMCLIB_BetaProjection3Ph_F32 ==
  pIn : Inport  OutDataTypeStr=Bus: SWLIBS_3Syst_F32  BusOutputAsStruct=on
  GMCLIB_BetaProjection3Ph_SF : S-Function  FunctionName=GMCLIB_BetaProjection3Ph_SF_F32  SFunctionDeploymentMode=off  EnableBusSupport=off
  copyright : Subsystem
      mask Display: text(10,90,'FILE:');text(10,75,'DESRIPTION:');text(10,60,'COPYRIGHT:');text(10,45,'VERSION:');text(10,30,'DATE:')
  copyright2 : Subsystem
      mask Display: text(10,90,'GMCLIB_BetaProjection3Ph_BAM_F32.slx');text(10,75,'3-phase Beta-projection transformation.');text(10,60,'NXP 2022');text(10,45,'1.0');text(10,30,'20-Apr-2022');
  pOut : Outport
  wires:
  GMCLIB_BetaProjection3Ph_SF/1 -> pOut/1
  pIn/1 -> GMCLIB_BetaProjection3Ph_SF/1

== system ammclib_bam_S32K3xx/GMCLIB/F32/GMCLIB_BetaProjection_F32 ==
  pIn : Inport  OutDataTypeStr=Bus: SWLIBS_3Syst_F32  BusOutputAsStruct=on
  GMCLIB_BetaProjection_SF : S-Function  FunctionName=GMCLIB_BetaProjection_SF_F32  SFunctionDeploymentMode=off  EnableBusSupport=off
  copyright : Subsystem
      mask Display: text(10,90,'FILE:');text(10,75,'DESRIPTION:');text(10,60,'COPYRIGHT:');text(10,45,'VERSION:');text(10,30,'DATE:')
  copyright2 : Subsystem
      mask Display: text(10,90,'GMCLIB_BetaProjection_BAM_F32.slx');text(10,75,'Beta Projection transformation.');text(10,60,'NXP 2022');text(10,45,'1.0');text(10,30,'20-Apr-2022');
  pOut : Outport
  wires:
  GMCLIB_BetaProjection_SF/1 -> pOut/1
  pIn/1 -> GMCLIB_BetaProjection_SF/1

== system ammclib_bam_S32K3xx/GMCLIB/F32/GMCLIB_Clark6Ph_F32 ==
  pIn : Inport  OutDataTypeStr=Bus: SWLIBS_6Syst_F32  BusOutputAsStruct=on
  GMCLIB_Clark6Ph_SF : S-Function  FunctionName=GMCLIB_Clark6Ph_SF_F32  Parameters=f32WindingShift  SFunctionDeploymentMode=off  EnableBusSupport=off
  copyright : Subsystem
      mask Display: text(10,90,'FILE:');text(10,75,'DESRIPTION:');text(10,60,'COPYRIGHT:');text(10,45,'VERSION:');text(10,30,'DATE:')
  copyright2 : Subsystem
      mask Display: text(10,90,'GMCLIB_Clark6Ph_BAM_F32.slx');text(10,75,'Direct 6-phase Clark transformation.');text(10,60,'NXP 2022');text(10,45,'1.0');text(10,30,'20-Apr-2022');
  pOut : Outport
  wires:
  GMCLIB_Clark6Ph_SF/1 -> pOut/1
  pIn/1 -> GMCLIB_Clark6Ph_SF/1

== system ammclib_bam_S32K3xx/GMCLIB/F32/GMCLIB_ClarkInv6Ph_F32 ==
  pIn : Inport  OutDataTypeStr=Bus: SWLIBS_2Syst_F32  BusOutputAsStruct=on
  GMCLIB_ClarkInv6Ph_SF : S-Function  FunctionName=GMCLIB_ClarkInv6Ph_SF_F32  Parameters=f32WindingShift  SFunctionDeploymentMode=off  EnableBusSupport=off
  copyright : Subsystem
      mask Display: text(10,90,'FILE:');text(10,75,'DESRIPTION:');text(10,60,'COPYRIGHT:');text(10,45,'VERSION:');text(10,30,'DATE:')
  copyright2 : Subsystem
      mask Display: text(10,90,'GMCLIB_ClarkInv6Ph_BAM_F32.slx');text(10,75,'Inverse Clarke transform for six-phase systems.');text(10,60,'NXP 2022');text(10,45,'1.0');text(10,30,'20-Apr-2022');
  pOut : Outport
  wires:
  GMCLIB_ClarkInv6Ph_SF/1 -> pOut/1
  pIn/1 -> GMCLIB_ClarkInv6Ph_SF/1

== system ammclib_bam_S32K3xx/GMCLIB/F32/GMCLIB_ClarkInv_F32 ==
  pIn : Inport  OutDataTypeStr=Bus: SWLIBS_2Syst_F32  BusOutputAsStruct=on
  GMCLIB_ClarkInv_SF : S-Function  FunctionName=GMCLIB_ClarkInv_SF_F32  SFunctionDeploymentMode=off  EnableBusSupport=off
  copyright : Subsystem
      mask Display: text(10,90,'FILE:');text(10,75,'DESRIPTION:');text(10,60,'COPYRIGHT:');text(10,45,'VERSION:');text(10,30,'DATE:')
  copyright2 : Subsystem
      mask Display: text(10,90,'GMCLIB_ClarkInv_BAM_F32.slx');text(10,75,'Inverse Clarke transformation');text(10,60,'NXP 2022');text(10,45,'1.0');text(10,30,'20-Apr-2022');
  pOut : Outport
  wires:
  GMCLIB_ClarkInv_SF/1 -> pOut/1
  pIn/1 -> GMCLIB_ClarkInv_SF/1

== system ammclib_bam_S32K3xx/GMCLIB/F32/GMCLIB_Clark_F32 ==
  pIn : Inport  OutDataTypeStr=Bus: SWLIBS_3Syst_F32  BusOutputAsStruct=on
  GMCLIB_Clark_SF : S-Function  FunctionName=GMCLIB_Clark_SF_F32  SFunctionDeploymentMode=off  EnableBusSupport=off
  copyright : Subsystem
      mask Display: text(10,90,'FILE:');text(10,75,'DESRIPTION:');text(10,60,'COPYRIGHT:');text(10,45,'VERSION:');text(10,30,'DATE:')
  copyright2 : Subsystem
      mask Display: text(10,90,'GMCLIB_Clark_BAM_F32.slx');text(10,75,'Clarke transformation.');text(10,60,'NXP 2022');text(10,45,'1.0');text(10,30,'20-Apr-2022');
  pOut : Outport
  wires:
  GMCLIB_Clark_SF/1 -> pOut/1
  pIn/1 -> GMCLIB_Clark_SF/1

== system ammclib_bam_S32K3xx/GMCLIB/F32/GMCLIB_DecouplingPMSM_F32 ==
  pUdq : Inport  OutDataTypeStr=Bus: SWLIBS_2Syst_F32  BusOutputAsStruct=on
  pIdq : Inport  Port=2  OutDataTypeStr=Bus: SWLIBS_2Syst_F32  BusOutputAsStruct=on
  f32AngularVel : Inport  Port=3  OutDataTypeStr=int32
  GMCLIB_DecouplingPMSM_SF : S-Function  FunctionName=GMCLIB_DecouplingPMSM_SF_F32  Parameters=showStates,f32Kd,s16KdShift,f32Kq,s16KqShift  SFunctionDeploymentMode=off  EnableBusSupport=off
  copyright : Subsystem
      mask Display: text(10,90,'FILE:');text(10,75,'DESRIPTION:');text(10,60,'COPYRIGHT:');text(10,45,'VERSION:');text(10,30,'DATE:')
  copyright2 : Subsystem
      mask Display: text(10,90,'GMCLIB_DecouplingPMSM_BAM_F32.slx');text(10,75,'Decoupling of d and q axis of PMSM model.');text(10,60,'NXP 2022');text(10,45,'1.0');text(10,30,'20-Apr-2022');
  f32Kd : Ground
  f32Kq : Ground
  s16KdShift : Ground
  s16KqShift : Ground
  pUdqDec : Outport
  wires:
  GMCLIB_DecouplingPMSM_SF/1 -> pUdqDec/1
  s16KqShift/1 -> GMCLIB_DecouplingPMSM_SF/7
  f32Kq/1 -> GMCLIB_DecouplingPMSM_SF/6
  s16KdShift/1 -> GMCLIB_DecouplingPMSM_SF/5
  f32Kd/1 -> GMCLIB_DecouplingPMSM_SF/4
  f32AngularVel/1 -> GMCLIB_DecouplingPMSM_SF/3
  pIdq/1 -> GMCLIB_DecouplingPMSM_SF/2
  pUdq/1 -> GMCLIB_DecouplingPMSM_SF/1

== system ammclib_bam_S32K3xx/GMCLIB/F32/GMCLIB_ElimDcBusRip_F32 ==
  pIn : Inport  OutDataTypeStr=Bus: SWLIBS_2Syst_F32  BusOutputAsStruct=on
  f32ArgDcBusMsr : Inport  Port=2  OutDataTypeStr=int32
  GMCLIB_ElimDcBusRip_SF : S-Function  FunctionName=GMCLIB_ElimDcBusRip_SF_F32  Parameters=showStates,f32ModIndex  SFunctionDeploymentMode=off  EnableBusSupport=off
  copyright : Subsystem
      mask Display: text(10,90,'FILE:');text(10,75,'DESRIPTION:');text(10,60,'COPYRIGHT:');text(10,45,'VERSION:');text(10,30,'DATE:')
  copyright2 : Subsystem
      mask Display: text(10,90,'GMCLIB_ElimDcBusRip_BAM_F32.slx');text(10,75,'DC Bus voltage ripple elimination function.');text(10,60,'NXP 2022');text(10,45,'1.0');text(10,30,'20-Apr-2022');
  f32ModIndex : Ground
  pOut : Outport
  wires:
  GMCLIB_ElimDcBusRip_SF/1 -> pOut/1
  f32ModIndex/1 -> GMCLIB_ElimDcBusRip_SF/3
  f32ArgDcBusMsr/1 -> GMCLIB_ElimDcBusRip_SF/2
  pIn/1 -> GMCLIB_ElimDcBusRip_SF/1

== system ammclib_bam_S32K3xx/GMCLIB/F32/GMCLIB_ParkInv_F32 ==
  pInAngle : Inport  OutDataTypeStr=Bus: SWLIBS_2Syst_F32  BusOutputAsStruct=on
  pIn : Inport  Port=2  OutDataTypeStr=Bus: SWLIBS_2Syst_F32  BusOutputAsStruct=on
  GMCLIB_ParkInv_SF : S-Function  FunctionName=GMCLIB_ParkInv_SF_F32  SFunctionDeploymentMode=off  EnableBusSupport=off
  copyright : Subsystem
      mask Display: text(10,90,'FILE:');text(10,75,'DESRIPTION:');text(10,60,'COPYRIGHT:');text(10,45,'VERSION:');text(10,30,'DATE:')
  copyright2 : Subsystem
      mask Display: text(10,90,'GMCLIB_ParkInv_BAM_F32.slx');text(10,75,'Inverse Park transformation.');text(10,60,'NXP 2022');text(10,45,'1.0');text(10,30,'20-Apr-2022');
  pOut : Outport
  wires:
  GMCLIB_ParkInv_SF/1 -> pOut/1
  pIn/1 -> GMCLIB_ParkInv_SF/2
  pInAngle/1 -> GMCLIB_ParkInv_SF/1

== system ammclib_bam_S32K3xx/GMCLIB/F32/GMCLIB_Park_F32 ==
  pInAngle : Inport  OutDataTypeStr=Bus: SWLIBS_2Syst_F32  BusOutputAsStruct=on
  pIn : Inport  Port=2  OutDataTypeStr=Bus: SWLIBS_2Syst_F32  BusOutputAsStruct=on
  GMCLIB_Park_SF : S-Function  FunctionName=GMCLIB_Park_SF_F32  SFunctionDeploymentMode=off  EnableBusSupport=off
  copyright : Subsystem
      mask Display: text(10,90,'FILE:');text(10,75,'DESRIPTION:');text(10,60,'COPYRIGHT:');text(10,45,'VERSION:');text(10,30,'DATE:')
  copyright2 : Subsystem
      mask Display: text(10,90,'GMCLIB_Park_BAM_F32.slx');text(10,75,'Park transformation.');text(10,60,'NXP 2022');text(10,45,'1.0');text(10,30,'20-Apr-2022');
  pOut : Outport
  wires:
  GMCLIB_Park_SF/1 -> pOut/1
  pIn/1 -> GMCLIB_Park_SF/2
  pInAngle/1 -> GMCLIB_Park_SF/1

== system ammclib_bam_S32K3xx/GMCLIB/F32/GMCLIB_PwmIct_F32 ==
  pIn : Inport  OutDataTypeStr=Bus: SWLIBS_2Syst_F32  BusOutputAsStruct=on
  GMCLIB_PwmIct_SF : S-Function  FunctionName=GMCLIB_PwmIct_SF_F32  SFunctionDeploymentMode=off  EnableBusSupport=off
  copyright : Subsystem
      mask Display: text(10,90,'FILE:');text(10,75,'DESRIPTION:');text(10,60,'COPYRIGHT:');text(10,45,'VERSION:');text(10,30,'DATE:')
  copyright2 : Subsystem
      mask Display: text(10,90,'GMCLIB_PwmIct_BAM_F32.slx');text(10,75,'General Sinusoidal PWM.');text(10,60,'NXP 2022');text(10,45,'1.0');text(10,30,'20-Apr-2022');
  u32Sector : Outport
  pOut : Outport  Port=2
  wires:
  GMCLIB_PwmIct_SF/2 -> pOut/1
  GMCLIB_PwmIct_SF/1 -> u32Sector/1
  pIn/1 -> GMCLIB_PwmIct_SF/1

== system ammclib_bam_S32K3xx/GMCLIB/F32/GMCLIB_SvmSci_F32 ==
  pIn : Inport  OutDataTypeStr=Bus: SWLIBS_2Syst_F32  BusOutputAsStruct=on
  GMCLIB_SvmSci_SF : S-Function  FunctionName=GMCLIB_SvmSci_SF_F32  SFunctionDeploymentMode=off  EnableBusSupport=off
  copyright : Subsystem
      mask Display: text(10,90,'FILE:');text(10,75,'DESRIPTION:');text(10,60,'COPYRIGHT:');text(10,45,'VERSION:');text(10,30,'DATE:')
  copyright2 : Subsystem
      mask Display: text(10,90,'GMCLIB_SvmSci_BAM_F32.slx');text(10,75,'General Sinusoidal Modulation with Injection of Third Harmonic.');text(10,60,'NXP 2022');text(10,45,'1.0');text(10,30,'20-Apr-2022');
  u32Sector : Outport
  pOut : Outport  Port=2
  wires:
  GMCLIB_SvmSci_SF/2 -> pOut/1
  GMCLIB_SvmSci_SF/1 -> u32Sector/1
  pIn/1 -> GMCLIB_SvmSci_SF/1

== system ammclib_bam_S32K3xx/GMCLIB/F32/GMCLIB_SvmStd6Ph_F32 ==
  pIn : Inport  OutDataTypeStr=Bus: SWLIBS_2Syst_F32  BusOutputAsStruct=on
  GMCLIB_SvmStd6Ph_SF : S-Function  FunctionName=GMCLIB_SvmStd6Ph_SF_F32  Parameters=f32WindingShift  SFunctionDeploymentMode=off  EnableBusSupport=off
  copyright : Subsystem
      mask Display: text(10,90,'FILE:');text(10,75,'DESRIPTION:');text(10,60,'COPYRIGHT:');text(10,45,'VERSION:');text(10,30,'DATE:')
  copyright2 : Subsystem
      mask Display: text(10,90,'GMCLIB_SvmStd6Ph_BAM_F32.slx');text(10,75,'Six-phase Space Vector Modulation.');text(10,60,'NXP 2022');text(10,45,'1.0');text(10,30,'20-Apr-2022');
  pOut : Outport
  pOutSector : Outport  Port=2
  wires:
  GMCLIB_SvmStd6Ph_SF/2 -> pOutSector/1
  GMCLIB_SvmStd6Ph_SF/1 -> pOut/1
  pIn/1 -> GMCLIB_SvmStd6Ph_SF/1

== system ammclib_bam_S32K3xx/GMCLIB/F32/GMCLIB_SvmStd_F32 ==
  pIn : Inport  OutDataTypeStr=Bus: SWLIBS_2Syst_F32  BusOutputAsStruct=on
  GMCLIB_SvmStd_SF : S-Function  FunctionName=GMCLIB_SvmStd_SF_F32  SFunctionDeploymentMode=off  EnableBusSupport=off
  copyright : Subsystem
      mask Display: text(10,90,'FILE:');text(10,75,'DESRIPTION:');text(10,60,'COPYRIGHT:');text(10,45,'VERSION:');text(10,30,'DATE:')
  copyright2 : Subsystem
      mask Display: text(10,90,'GMCLIB_SvmStd_BAM_F32.slx');text(10,75,'Standard Space Vector Modulation.');text(10,60,'NXP 2022');text(10,45,'1.0');text(10,30,'20-Apr-2022');
  u32Sector : Outport
  pOut : Outport  Port=2
  wires:
  GMCLIB_SvmStd_SF/2 -> pOut/1
  GMCLIB_SvmStd_SF/1 -> u32Sector/1
  pIn/1 -> GMCLIB_SvmStd_SF/1
